simulink model "impedance"  (Simulink 7.4)
settings: Solver=ode45  StartTime=0.0  StopTime=8  MinStep=0.01  RelTol=1e-3
values from neighbouring files (symbols this model uses):
  Kd = Kp.^0.5*2    [WAMforcecontrol.m]    (also in batchwamobs.m = 50*eye(7); paralelcontrol2R.m = eye(n)*1000)
  Kp = 25*eye(7)    [batchwamobs.m]    (also in paralelcontrol2R.m = eye(n)*2500)
undefined symbols (not defined in the file or in its folder): jacobderivblock, Kimp, model1, model2, model3, model4, model5, model6, ncalculest, p560, T2screw
libraries: roblocks x3
settings Model: Creator=acolome  LastModifiedBy=acolome

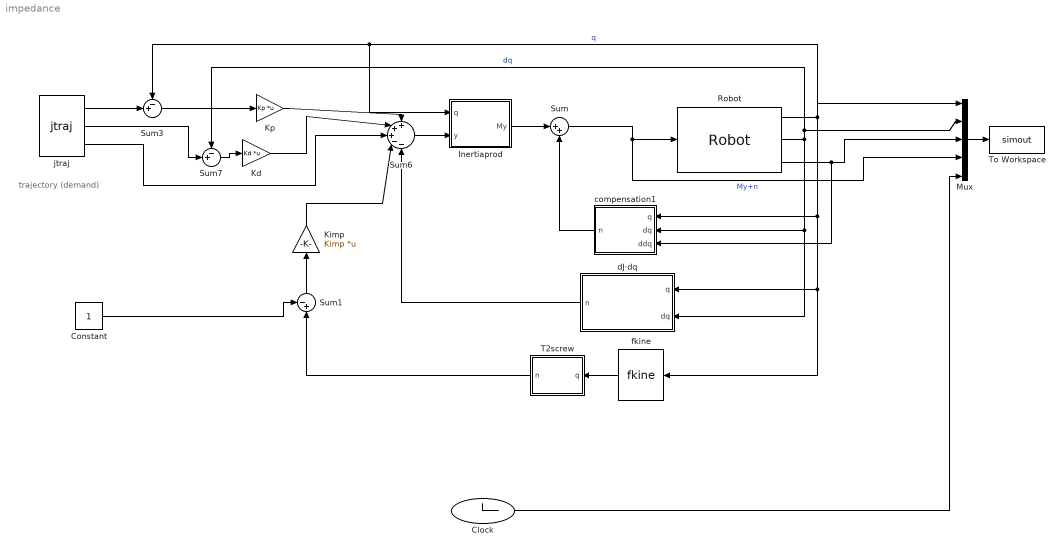
== system impedance ==
  note: trajectory
      | (demand)
  Clock : Clock
      settings: Decimation=100
  Constant : Constant  OutDataType=fixdt(1, 16)  OutScaling=2^0
  Inertiaprod : Subsystem  mask{robot=p560, g=[0 0 9.81]}
      mask prompts: robot "Robot Object"; g "Gravity"
      mask init:
      | n=robot.n
      mask Display:
      | port_label('output',1,'M(q)y')
      | 
      | port_label('input', 1, 'q')
      | port_label('input', 2, 'y')
  Kd : Gain  Gain=Kd  Multiplication=Matrix(K*u)  SaturateOnIntegerOverflow=on  OutDataTypeStr=Inherit: Same as input  ParamDataTypeStr=Inherit: Same as input
  Kimp : Gain  Gain=Kimp  Multiplication=Matrix(K*u)  SaturateOnIntegerOverflow=on  OutDataTypeStr=Inherit: Same as input  ParamDataTypeStr=Inherit: Same as input
  Kp : Gain  Gain=Kp  Multiplication=Matrix(K*u)  SaturateOnIntegerOverflow=on  OutDataTypeStr=Inherit: Same as input  ParamDataTypeStr=Inherit: Same as input
  Mux : Mux  Inputs=5
  Robot : roblocks/Robot  SystemSampleTime=-1  robot=p560  q0=[0 0 0 0 0 pi/20]*0
      link override Integrator1: InitialCondition=q0
  Sum : Sum  Inputs=|++  OutDataType=fixdt(1, 16)  OutScaling=2^0
  Sum1 : Sum  Inputs=-+|  SaturateOnIntegerOverflow=on  InputSameDT=on  OutDataTypeStr=Inherit: Same as first input
  Sum3 : Sum  Inputs=-+|  SaturateOnIntegerOverflow=on  InputSameDT=on  OutDataTypeStr=Inherit: Same as first input
  Sum6 : Sum  Inputs=+++--  OutDataType=fixdt(1, 16)  OutScaling=2^0
  Sum7 : Sum  Inputs=-+|  SaturateOnIntegerOverflow=on  InputSameDT=on  OutDataTypeStr=Inherit: Same as first input
  T2screw : Subsystem  mask{robot=p560}
      mask prompts: robot "Robot Object"
      mask init:
      | n=robot.n
      mask Display:
      | port_label('output',1,'xe')
      | 
      | port_label('input', 1, 'T')
  To Workspace : ToWorkspace  VariableName=simout  SampleTime=-1  SaveFormat=Array
  compensation1 : Subsystem  mask{robot=p560, g=[0 0 9.81], model1=model1, model2=model2, model3=model3, model4=model4, model5=model5, model6=model6}
      mask prompts: robot "Robot Object"; g "Gravity"; model1 "n1"; model2 "n2"; model3 "n3"; model4 "n4"; model5 "n5"; model6 "n6"
      mask init:
      | n=robot.n
      mask Display:
      | port_label('output',1,'n(q,dq)')
      | 
      | port_label('input', 1, 'q')
      | port_label('input', 2, 'dq')
      | port_label('input', 3, 'ddq')
  dJ·dq : Subsystem  mask{robot=p560, g=[0 0 9.81], model1=model1, model2=model2, model3=model3, model4=model4, model5=model5, model6=model6}
      mask prompts: robot "Robot Object"; g "Gravity"; model1 "n1"; model2 "n2"; model3 "n3"; model4 "n4"; model5 "n5"; model6 "n6"
      mask init:
      | n=robot.n
      mask Display:
      | port_label('output',1,'dJ(q,dq)·dq')
      | 
      | port_label('input', 1, 'q')
      | port_label('input', 2, 'dq')
  fkine : roblocks/fkine  SystemSampleTime=-1  robot=p560
  jtraj : roblocks/jtraj  SystemSampleTime=-1  q0=[0 0 0 0 0 pi/20]*0  qf=[1 1 1 1 1 1]  tmax=8
      link override MATLAB Fcn: MATLABFcn=squeeze(interp1(t,q,u))
      link override MATLAB Fcn1: MATLABFcn=squeeze(interp1(t,qd,u))
      link override MATLAB Fcn2: MATLABFcn=squeeze(interp1(t,qdd,u))
  wires:
  Mux/1 -> To Workspace/1
  jtraj/2 -> Sum7/2
  Sum7/1 -> Kd/1
  Sum3/1 -> Kp/1
  jtraj/3 -> Sum6/3
  Kd/1 -> Sum6/2
  Kp/1 -> Sum6/1
  jtraj/1 -> Sum3/2
  Robot/1 -> Sum3/1, Inertiaprod/1(q), Mux/1, compensation1/1(q), dJ·dq/1(q), fkine/1  "q"
  Robot/2 -> Sum7/1, Mux/2, compensation1/2(dq), dJ·dq/2(dq)  "dq"
  Sum6/1 -> Inertiaprod/2(y)
  Robot/3 -> Mux/3, compensation1/3(ddq)
  Clock/1 -> Mux/5
  compensation1/1(n) -> Sum/2
  Inertiaprod/1(My) -> Sum/1
  Sum/1 -> Robot/1, Mux/4  "My+n"
  dJ·dq/1(n) -> Sum6/5
  fkine/1 -> T2screw/1(q)
  T2screw/1(n) -> Sum1/2
  Constant/1 -> Sum1/1
  Kimp/1 -> Sum6/4
  Sum1/1 -> Kimp/1

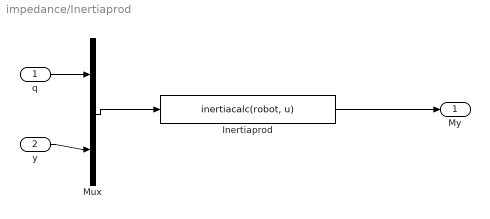
== system impedance/Inertiaprod ==
  q : Inport  OutDataType=fixdt(1, 16)  OutScaling=2^0
  y : Inport  Port=2  OutDataType=fixdt(1, 16)  OutScaling=2^0
  Inertiaprod : MATLABFcn  MATLABFcn=inertiacalc(robot, u)  OutputDimensions=n
  Mux : Mux  Inputs=2
  My : Outport  OutDataType=fixdt(1, 16)  OutScaling=2^0
  wires:
  Mux/1 -> Inertiaprod/1
  q/1 -> Mux/1
  Inertiaprod/1 -> My/1
  y/1 -> Mux/2

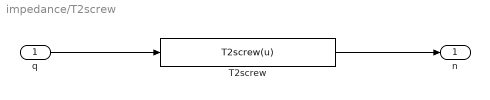
== system impedance/T2screw ==
  q : Inport  OutDataType=fixdt(1, 16)  OutScaling=2^0
  T2screw : MATLABFcn  MATLABFcn=T2screw(u)  OutputDimensions=6
  n : Outport  OutDataType=fixdt(1, 16)  OutScaling=2^0
  wires:
  T2screw/1 -> n/1
  q/1 -> T2screw/1

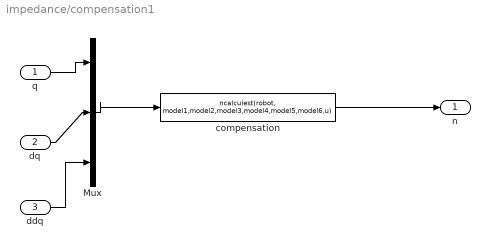
== system impedance/compensation1 ==
  q : Inport  OutDataType=fixdt(1, 16)  OutScaling=2^0
  dq : Inport  Port=2  OutDataType=fixdt(1, 16)  OutScaling=2^0
  ddq : Inport  Port=3  OutDataType=fixdt(1, 16)  OutScaling=2^0
  Mux : Mux  Inputs=3
  compensation : MATLABFcn  MATLABFcn=ncalculest(robot, model1,model2,model3,model4,model5,model6,u)  OutputDimensions=n
  n : Outport  OutDataType=fixdt(1, 16)  OutScaling=2^0
  wires:
  Mux/1 -> compensation/1
  q/1 -> Mux/1
  compensation/1 -> n/1
  dq/1 -> Mux/2
  ddq/1 -> Mux/3

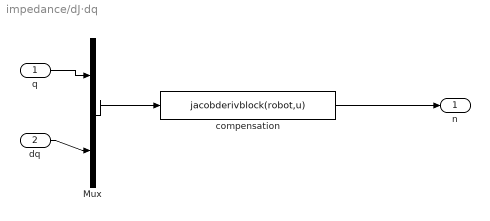
== system impedance/dJ·dq ==
  q : Inport  OutDataType=fixdt(1, 16)  OutScaling=2^0
  dq : Inport  Port=2  OutDataType=fixdt(1, 16)  OutScaling=2^0
  Mux : Mux  Inputs=2
  compensation : MATLABFcn  MATLABFcn=jacobderivblock(robot,u)  OutputDimensions=n
  n : Outport  OutDataType=fixdt(1, 16)  OutScaling=2^0
  wires:
  Mux/1 -> compensation/1
  q/1 -> Mux/1
  compensation/1 -> n/1
  dq/1 -> Mux/2
